simulink model "PSlabexp3_19EE30018"  (R2021a)
settings: Solver=VariableStepAuto  StartTime=0.0  StopTime=inf  RelTol=1e-3
libraries: spsVoltageMeasurementLib x8, spsRMSLib x7, simulink x5, spsGroundLib x4, spsFourierLib x2, spsabctoAlphaBetaZeroLib x2, spsCurrentMeasurementLib x2, spsControlledVoltageSourceLib x2, spsThreePhaseProgrammableVoltageSourceLib x1, spsDCMachineLib x1, spsPower3phInstantaneousLib x1, spsSimplifiedSynchronousMachineSIUnitsLib x1
settings Model: Creator=win10  LastModifiedBy=mansi
settings SolverCC: ZeroCrossAlgorithm=Adaptive
settings DebuggingCC: IgnoredZcDiagnostic=none

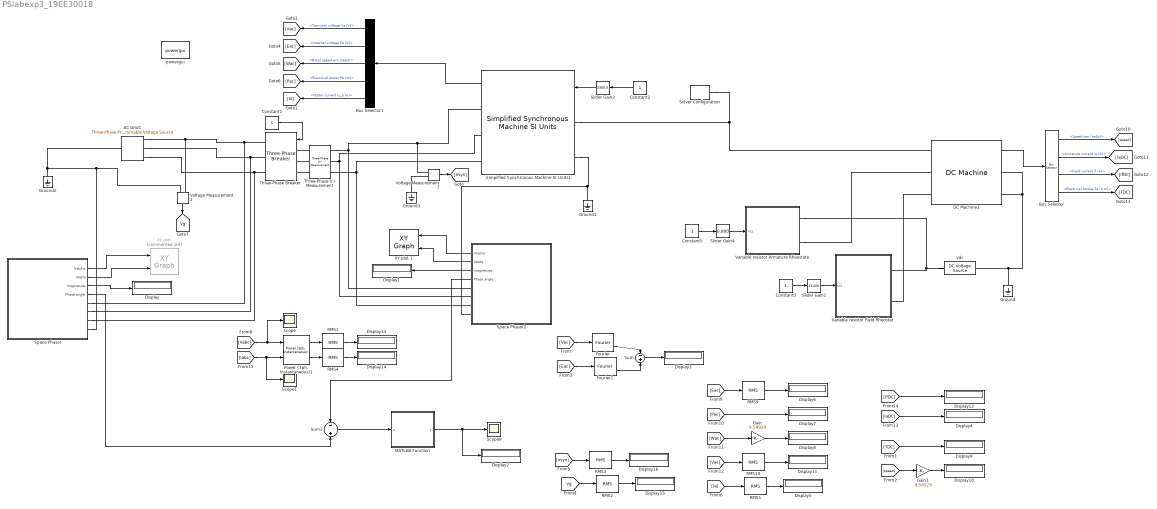
== system PSlabexp3_19EE30018 ==
  AC Grid1 : spsThreePhaseProgrammableVoltageSourceLib/Three-Phase Programmable Voltage Source  PositiveSequence="[3300  0 50.01]"  VariationEntity=None  VariationType=Step  VariationTypeAlt=Step  VariationStep=0.5  VariationRate=10  VariationMagnitude=0.3  VariationFrequency=2  VariationTiming=[1 2]  VariationPhaseA=off  Amplitudes=[1 0.8 1.2 1.0]  TimeValues=[0 0.1 0.15 0.2]  HarmonicGeneration=off  HarmonicA=[3 0.2 -25 0]  HarmonicB=[2 0.15 35 2]  Timing="[0.05  3]"  BusType=swing  Pref=0  Qref=0  Qmin=-inf  Qmax=inf
  Bus Selector : BusSelector  OutputSignals=Speed wm (rad/s),Armature current ia (A),Field current if (A),Electrical torque Te (n m)
  Bus Selector1 : BusSelector  OutputSignals=Terminal voltage Va (V),Internal voltage Ea (V),Rotor speed wm (rad/s),Electrical power Pe (W),Stator current is_a (A)
  Constant{1..3,5} (4 alike) : Constant
  DC Machine1 : spsDCMachineLib/DC Machine  PresetModel=22: 225HP 500V 1750RPM Field:300V  MechanicalLoad=Mechanical rotational port  FieldType=Wound  ShowDetailedParameters=on  MeasurementBus=off  RLa=[0.07571 0.001986]  RLf=[33.46 3.499]  Laf=0.2874  MachineConstant=Torque constant (N.m/A)  Ke=1.8  Kt=1.8  J=0.9177  Bm=0.02289  Tf=23.81  w0=0  Ifinit=14.9432157800359  TsPowergui=0  TsBlock=-1
  Display{,1..16} (17 alike) : Display
  Fourier : spsFourierLib/Fourier  Freq=50  n=1  InInit=[0, 0]  Ts=0
      settings: SourceProductBaseCode=PS
  Fourier1 : spsFourierLib/Fourier  Freq=50  n=1  InInit=[0, 0]  Ts=0
      settings: SourceProductBaseCode=PS
  Gain : Gain  Gain=9.54929
  Gain1 : Gain  Gain=9.54929
  Ground{,1..3} (4 alike) : spsGroundLib/Ground  LConnTagsString=a
  MATLAB Function : MATLAB Function  TreatAsAtomicUnit=on
  "Power (3ph, Instantaneous)1" : spsPower3phInstantaneousLib/Power (3ph, Instantaneous)
  RMS{1..5,9..10} (7 alike) : spsRMSLib/RMS  TrueRMS=on  Freq=50  RMSInit=0  Ts=0
  Scope : Scope
  Scope1 : Scope
  Scope9 : Scope
  Simplified Synchronous Machine SI Units1 : spsSimplifiedSynchronousMachineSIUnitsLib/Simplified Synchronous Machine SI Units  ConnectionType=4-wire Y  MechanicalLoad=Mechanical rotational port  MeasurementBus=off  NominalParameters=[0.2e6 3300 50]  Mechanical=[24.1370 65 2]  InternalRL=[10 0.3466]  InitialConditions="[-99,0   0,0,0   0,-120,120 ]"  IterativeDiscreteModel=Trapezoidal non iterative  TsBlock=-1  TsPowergui=0  LoadFlowParameters=[1,0,0,0,0]  Units=1  BusType=PQ  Pref=0.05e6  Qref=0.05e6  Qmin=-inf  Qmax=+inf  PLF=0  QLF=0
      settings: SourceProductBaseCode=PS
  Slider Gain1 : simulink/Math Operations/Slider Gain  gain=13.050  low=5  high=40
  Slider Gain2 : simulink/Math Operations/Slider Gain  gain=3300.0  low=0  high=3300
  Slider Gain4 : simulink/Math Operations/Slider Gain  gain=0.800  low=0.0001  high=20
  Solver Configuration : nesl_utility/Solver Configuration  PhysicalDomain=network_engine_domain  SubClassName=solver  LeftPortType=input  RightPortType=generic  Tones=[]  Harmonics=[]  SimulateNoise=off  Profile=off  UseLocalSampling=off  EnableSwitchedLinearOptims=on  FrequencyDomain=off  UseCCode=off  RelTol=0.001  AbsTol=1e-06  MinStep=1e-09  ToWorkspace=off  RevertToSquareIcSolve=off  NumHomotopyIterations=100  PhasorMode=off  PhasorModeNumHarmonics=1  DoDC=off  ResidualTolerance=1e-09  UseLocalSolver=off  LocalSolverChoice=NE_BACKWARD_EULER_ADVANCER  LocalSolverSampleTime=0.001  DoFixedCost=off  MaxNonlinIter=3  MaxModeIter=2  ComputeImpulses=off  ImpulseIterations=2  LinearAlgebra=Sparse  EquationFormulation=NE_TIME_EF  DelaysMemoryBudget=1024  AutomaticFiltering=on  FilteringTimeConstant=0.001  PartitionStorageMethod=AS_NEEDED  PartitionMemoryBudget=1024  PartitionMethod=FAST
  Space Phasor : Subsystem
  Space Phasor2 : Subsystem
  Sum : Sum  Inputs=-+
  Sum3 : Sum  Inputs=-+  InputSameDT=on  SaturateOnIntegerOverflow=on  OutDataTypeStr=Inherit: Same as first input
  Three-Phase V-I Measurement : spsThreePhaseVIMeasurementLib/Three-Phase V-I Measurement  VoltageMeasurement=phase-to-ground  SetLabelV=on  LabelV=Vabc  Vpu=off  VpuLL=off  CurrentMeasurement=yes  SetLabelI=on  LabelI=Iabc  Ipu=off  Pbase=100e6  Vbase=500e3  OutputType=Complex  PhasorSimulation=off  PSBequivalent=0
  Three-Phase Breaker : spsThreePhaseBreakerLib/Three-Phase Breaker  InitialState=open  SwitchA=on  SwitchB=on  SwitchC=on  SwitchTimes=[0.1]  External=on  BreakerResistance=0.001  SnubberResistance=1e6  SnubberCapacitance=inf  Measurements=None
  Variable resistor Armature Rheostate : Subsystem
  Variable resistor Field Rheostat : Subsystem
  Voltage Measurement2 : spsVoltageMeasurementLib/Voltage Measurement  PhasorSimulation=off  OutputType=Complex  PSBequivalent=0
  Voltage Measurement7 : spsVoltageMeasurementLib/Voltage Measurement  PhasorSimulation=off  OutputType=Complex  PSBequivalent=0
  "XY plot " : simulink/Sinks/XY Graph  Commented=on  xmin=-3000  xmax=3000  ymin=-3000  ymax=3000  st=-1
  XY plot 1 : simulink/Sinks/XY Graph  xmin=-3000  xmax=3000  ymin=-3000  ymax=3000  st=-1
  powergui : spspowerguiLib/powergui  Priority=1  SimulationMode=Continuous  SampleTime=1e-6  frequency=50  Iterations=50  frequencyindice=0  Pbase=100e6  ErrMax=1e-4  UnitsV=kV  UnitsW=MW  buscounter=0  FunctionMessages=off  echomessages=off  EnableUseOfTLC=off  CurrentSourceSwitches=off  DisableSnubberDevices=off  DisableRonSwitches=off  DisableVfSwitches=off  DisplayEquations=off  AutomaticDiscreteSolvers=off  SolverType=Tustin/Backward Euler (TBE)  Interpol=off  ExternalGateDelay=off  methode=off  Ts=100  x0status=blocks  SPID=on  SwTol=0  HookPort=off  NonlinearTolerance=1e-4  nMaxIteration=100  ContinueOnMaxIteration=off  RestoreLinks=warning  ResistiveCurrentMeasurement=off  Frange=[0:2:500]  Ylog=off  Xlog=on  ShowGrid=off  save=off  variable=ZData  structure=0  ZoomFFT=off  StartTime=0.0  cycles=1  DisplayStyle=1  fundamental=60  FreqAxis=off  MaxFrequency=1000  frequencyindicesteady=1  RmsSteady=1  display=off
  "vdc " : spsDCVoltageSourceLib/DC Voltage Source  Amplitude=500  Measurements=None
  tag scope: Vg=global
  wires:
  Slider Gain2/1 -> Simplified Synchronous Machine SI Units1/1
  MATLAB Function/1(y) -> Display2/1, Scope9/1
  Space Phasor2/3(magnetude) -> Display1/1
  Space Phasor2/2(Vbeta) -> XY plot 1/2
  Constant1/1 -> Three-Phase Breaker/1
  Sum3/1 -> MATLAB Function/1(u)
  Space Phasor/2(Vbeta) -> "XY plot "/2
  Space Phasor2/4(Phase angle) -> Sum3/1
  Space Phasor/3(magnetude) -> Display/1
  Space Phasor2/1(Valpha) -> XY plot 1/1
  Space Phasor/4(Phase angle) -> Sum3/2
  Space Phasor/1(Valpha) -> "XY plot "/1
  Voltage Measurement2/1 -> [Vg]
  Constant2/1 -> Slider Gain2/1
  Simplified Synchronous Machine SI Units1/1 -> Bus Selector1/1
  Bus Selector1/1 -> [Vac]  "<Terminal voltage Va (V)>"
  Bus Selector1/2 -> [Eac]  "<Internal voltage Ea (V)>"
  Bus Selector1/3 -> [Wac]  "<Rotor speed wm (rad/s)>"
  Bus Selector1/4 -> [Pac]  "<Electrical power Pe (W)>"
  Constant5/1 -> Slider Gain4/1
  Slider Gain1/1 -> Variable resistor Field Rheostat/1(In1)
  Constant3/1 -> Slider Gain1/1
  Slider Gain4/1 -> Variable resistor Armature Rheostate/1(In1)
  DC Machine1/1 -> Bus Selector/1
  Bus Selector/1 -> [speed]  "<Speed wm (rad/s)>"
  Bus Selector/2 -> [IaDC]  "<Armature current ia (A)>"
  Bus Selector/3 -> [IfDC]  "<Field current if (A)>"
  Bus Selector/4 -> [TDC]  "<Electrical torque Te (n m)>"
  Gain1/1 -> Display10/1
  [IfDC] -> Display12/1
  [IaDC] -> Display4/1
  [TDC] -> Display9/1
  [speed] -> Gain1/1
  RMS10/1 -> Display11/1
  [Eac] -> RMS9/1
  [Wac] -> Gain/1
  Gain/1 -> Display8/1
  [Vac] -> RMS10/1
  RMS9/1 -> Display6/1
  [Pac] -> Display7/1
  [Iabc] -> Scope1/1, "Power (3ph, Instantaneous)1"/2
  [Vabc] -> Scope/1, "Power (3ph, Instantaneous)1"/1
  [Vsyn] -> RMS3/1
  RMS3/1 -> Display16/1
  RMS2/1 -> Display15/1
  [Vg] -> RMS2/1
  Voltage Measurement7/1 -> [Vsyn]
  "Power (3ph, Instantaneous)1"/1 -> RMS1/1
  RMS1/1 -> Display13/1
  "Power (3ph, Instantaneous)1"/2 -> RMS4/1
  RMS4/1 -> Display14/1
  [Vac] -> Fourier/1
  [Eac] -> Fourier1/1
  Fourier/2 -> Sum/1
  Fourier1/2 -> Sum/2
  Sum/1 -> Display3/1
  Bus Selector1/5 -> [Ia]  "<Stator current is_a (A)>"
  [Ia] -> RMS5/1
  RMS5/1 -> Display5/1
  connections:
  Space Phasor/RConn3 -- AC Grid1/RConn3 -- Three-Phase Breaker/RConn3
  Space Phasor/RConn2 -- AC Grid1/RConn2 -- Three-Phase Breaker/RConn2
  Simplified Synchronous Machine SI Units1/RConn3 -- Space Phasor2/RConn3 -- Three-Phase V-I Measurement/RConn3
  Space Phasor2/RConn1 -- Three-Phase V-I Measurement/RConn1 -- Voltage Measurement7/LConn1 -- Simplified Synchronous Machine SI Units1/RConn1
  Ground2/LConn1 -- Space Phasor/RConn4 -- Voltage Measurement2/LConn2 -- AC Grid1/LConn1
  Space Phasor/RConn1 -- AC Grid1/RConn1 -- Voltage Measurement2/LConn1 -- Three-Phase Breaker/RConn1
  Space Phasor2/RConn4 -- Simplified Synchronous Machine SI Units1/LConn2 -- Ground1/LConn1
  Variable resistor Armature Rheostate/RConn1 -- Variable resistor Field Rheostat/RConn1 -- "vdc "/RConn1
  Simplified Synchronous Machine SI Units1/LConn1 -- DC Machine1/LConn1 -- Solver Configuration/RConn1
  DC Machine1/RConn2 -- DC Machine1/RConn1 -- Ground/LConn1 -- "vdc "/LConn1
  Variable resistor Field Rheostat/RConn2 -- DC Machine1/LConn3
  Variable resistor Armature Rheostate/RConn2 -- DC Machine1/LConn2
  Space Phasor2/RConn2 -- Three-Phase V-I Measurement/RConn2 -- Simplified Synchronous Machine SI Units1/RConn2
  Voltage Measurement7/LConn2 -- Ground3/LConn1
  Three-Phase V-I Measurement/LConn1 -- Three-Phase Breaker/LConn1
  Three-Phase V-I Measurement/LConn2 -- Three-Phase Breaker/LConn2
  Three-Phase V-I Measurement/LConn3 -- Three-Phase Breaker/LConn3

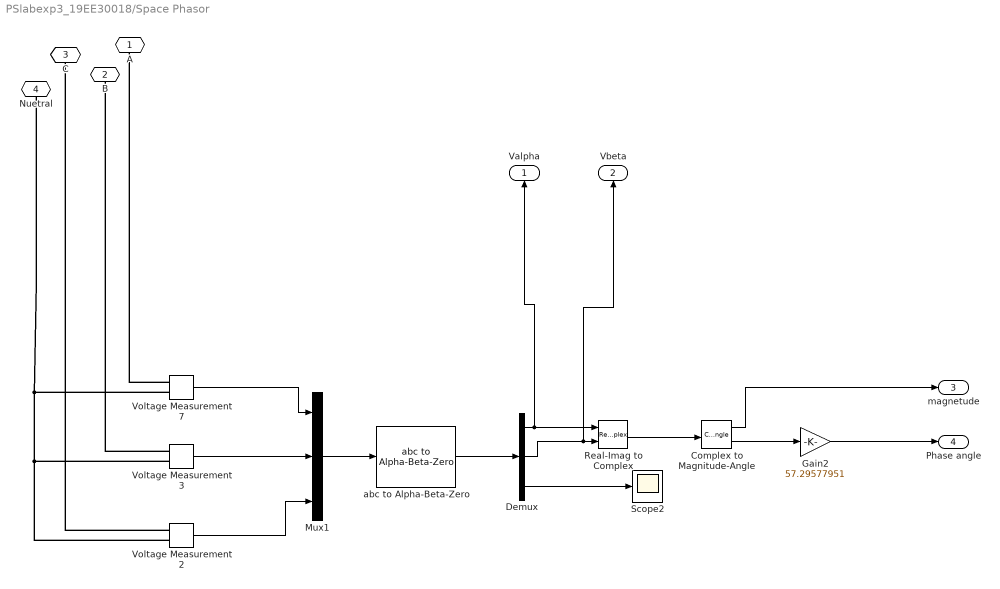
== system PSlabexp3_19EE30018/Space Phasor ==
  Complex to Magnitude-Angle : ComplexToMagnitudeAngle
  Demux : Demux  Outputs=3
  Gain2 : Gain  Gain=57.29577951
  Mux1 : Mux  Inputs=3
  Real-Imag to Complex : RealImagToComplex
  Scope2 : Scope
  Voltage Measurement2 : spsVoltageMeasurementLib/Voltage Measurement  PhasorSimulation=off  OutputType=Complex  PSBequivalent=0
  Voltage Measurement3 : spsVoltageMeasurementLib/Voltage Measurement  PhasorSimulation=off  OutputType=Complex  PSBequivalent=0
  Voltage Measurement7 : spsVoltageMeasurementLib/Voltage Measurement  PhasorSimulation=off  OutputType=Complex  PSBequivalent=0
  abc to Alpha-Beta-Zero : spsabctoAlphaBetaZeroLib/abc to Alpha-Beta-Zero
      settings: SourceProductBaseCode=PS
  A : PMIOPort  Side=Right
  B : PMIOPort  Port=2  Side=Right
  C : PMIOPort  Port=3  Side=Right
  Nuetral : PMIOPort  Port=4  Side=Right
  Valpha : Outport
  Vbeta : Outport  Port=2
  magnetude : Outport  Port=3
  Phase angle : Outport  Port=4
  wires:
  Complex to Magnitude-Angle/1 -> magnetude/1
  Real-Imag to Complex/1 -> Complex to Magnitude-Angle/1
  Demux/2 -> Vbeta/1, Real-Imag to Complex/2
  Demux/1 -> Valpha/1, Real-Imag to Complex/1
  Demux/3 -> Scope2/1
  abc to Alpha-Beta-Zero/1 -> Demux/1
  Voltage Measurement7/1 -> Mux1/1
  Mux1/1 -> abc to Alpha-Beta-Zero/1
  Complex to Magnitude-Angle/2 -> Gain2/1
  Voltage Measurement2/1 -> Mux1/3
  Gain2/1 -> Phase angle/1
  Voltage Measurement3/1 -> Mux1/2
  connections:
  Voltage Measurement2/LConn2 -- Voltage Measurement3/LConn2 -- Nuetral/RConn1 -- Voltage Measurement7/LConn2
  Voltage Measurement7/LConn1 -- A/RConn1
  Voltage Measurement2/LConn1 -- C/RConn1
  Voltage Measurement3/LConn1 -- B/RConn1

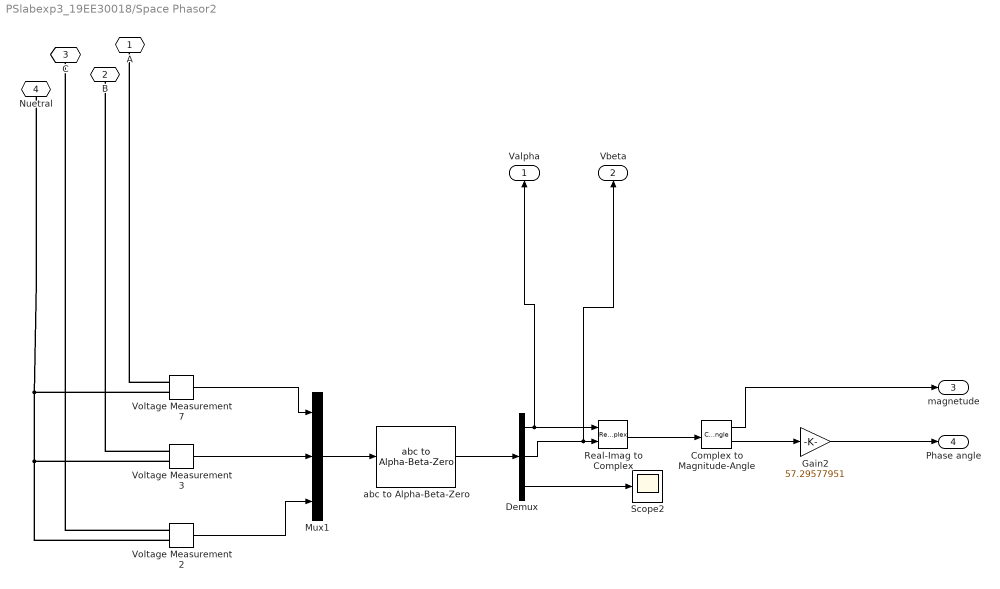
== system PSlabexp3_19EE30018/Space Phasor2 ==
  Complex to Magnitude-Angle : ComplexToMagnitudeAngle
  Demux : Demux  Outputs=3
  Gain2 : Gain  Gain=57.29577951
  Mux1 : Mux  Inputs=3
  Real-Imag to Complex : RealImagToComplex
  Scope2 : Scope
  Voltage Measurement2 : spsVoltageMeasurementLib/Voltage Measurement  PhasorSimulation=off  OutputType=Complex  PSBequivalent=0
  Voltage Measurement3 : spsVoltageMeasurementLib/Voltage Measurement  PhasorSimulation=off  OutputType=Complex  PSBequivalent=0
  Voltage Measurement7 : spsVoltageMeasurementLib/Voltage Measurement  PhasorSimulation=off  OutputType=Complex  PSBequivalent=0
  abc to Alpha-Beta-Zero : spsabctoAlphaBetaZeroLib/abc to Alpha-Beta-Zero
      settings: SourceProductBaseCode=PS
  A : PMIOPort  Side=Right
  B : PMIOPort  Port=2  Side=Right
  C : PMIOPort  Port=3  Side=Right
  Nuetral : PMIOPort  Port=4  Side=Right
  Valpha : Outport
  Vbeta : Outport  Port=2
  magnetude : Outport  Port=3
  Phase angle : Outport  Port=4
  wires:
  Complex to Magnitude-Angle/1 -> magnetude/1
  Real-Imag to Complex/1 -> Complex to Magnitude-Angle/1
  Demux/2 -> Vbeta/1, Real-Imag to Complex/2
  Demux/1 -> Valpha/1, Real-Imag to Complex/1
  Demux/3 -> Scope2/1
  abc to Alpha-Beta-Zero/1 -> Demux/1
  Voltage Measurement7/1 -> Mux1/1
  Mux1/1 -> abc to Alpha-Beta-Zero/1
  Complex to Magnitude-Angle/2 -> Gain2/1
  Voltage Measurement2/1 -> Mux1/3
  Gain2/1 -> Phase angle/1
  Voltage Measurement3/1 -> Mux1/2
  connections:
  Voltage Measurement2/LConn2 -- Voltage Measurement3/LConn2 -- Nuetral/RConn1 -- Voltage Measurement7/LConn2
  Voltage Measurement7/LConn1 -- A/RConn1
  Voltage Measurement2/LConn1 -- C/RConn1
  Voltage Measurement3/LConn1 -- B/RConn1

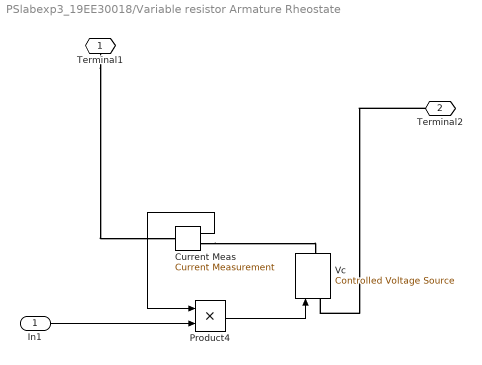
== system PSlabexp3_19EE30018/Variable resistor Armature Rheostate ==
  In1 : Inport
  Current Meas : spsCurrentMeasurementLib/Current Measurement  PhasorSimulation=off  OutputType=Complex  PSBequivalent=0
  Product4 : Product
  Vc : spsControlledVoltageSourceLib/Controlled Voltage Source  Initialize=on  Source_Type=DC  Amplitude=0  Phase=0  Frequency=0  Measurements=None
  Terminal1 : PMIOPort  Side=Right
  Terminal2 : PMIOPort  Port=2  Side=Right
  wires:
  Current Meas/1 -> Product4/1
  In1/1 -> Product4/2
  Product4/1 -> Vc/1
  connections:
  Terminal2/RConn1 -- Vc/LConn1
  Terminal1/RConn1 -- Current Meas/LConn1
  Current Meas/RConn1 -- Vc/RConn1

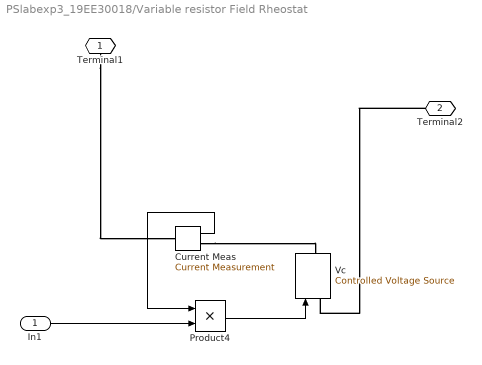
== system PSlabexp3_19EE30018/Variable resistor Field Rheostat ==
  In1 : Inport
  Current Meas : spsCurrentMeasurementLib/Current Measurement  PhasorSimulation=off  OutputType=Complex  PSBequivalent=0
  Product4 : Product
  Vc : spsControlledVoltageSourceLib/Controlled Voltage Source  Initialize=on  Source_Type=DC  Amplitude=0  Phase=0  Frequency=0  Measurements=None
  Terminal1 : PMIOPort  Side=Right
  Terminal2 : PMIOPort  Port=2  Side=Right
  wires:
  Current Meas/1 -> Product4/1
  In1/1 -> Product4/2
  Product4/1 -> Vc/1
  connections:
  Terminal2/RConn1 -- Vc/LConn1
  Terminal1/RConn1 -- Current Meas/LConn1
  Current Meas/RConn1 -- Vc/RConn1

== matlab function PSlabexp3_19EE30018/MATLAB Function ==
  data: u input; y output
function y = fcnphase(u)
%#codegen
y=u;
if u<0
y=360+u;
end
